simulink model "simulador_secador_solar"  (R2024b)
settings: Solver=VariableStepAuto  StartTime=0.0  StopTime=1000  RelTol=1e-3
values from neighbouring files (symbols this model uses):
  T_mu = 4.5    [G.mat]
settings Model: Creator=Celso  LastModifiedBy=Salvador

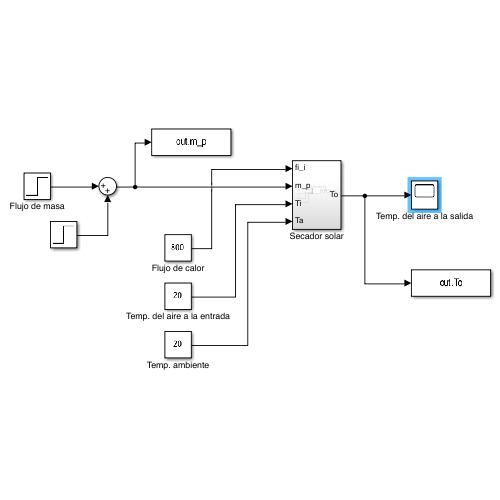
[thumbnail: Simulink's stored preview of the top-level diagram]
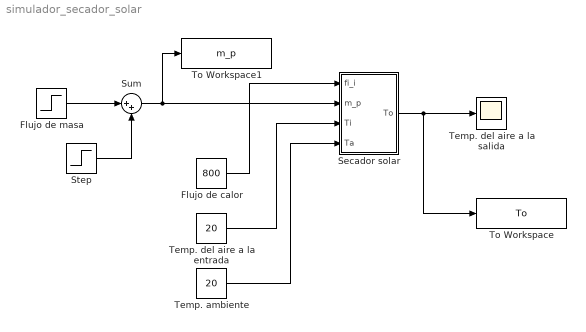
== system simulador_secador_solar ==
  Flujo de calor : Constant  Value=800
  Flujo de masa : Step  Time=0  After=0.02  SampleTime=0
  Secador solar : Subsystem
  Step : Step  Time=450  After=0.03  SampleTime=0
  Sum : Sum  Inputs=|++
  Temp. ambiente : Constant  Value=20
  Temp. del aire a la entrada : Constant  Value=20
  Temp. del aire a la salida : Scope
  To Workspace : ToWorkspace  VariableName=To  SampleTime=T_mu
  To Workspace1 : ToWorkspace  VariableName=m_p  SampleTime=T_mu
  wires:
  Temp. del aire a la entrada/1 -> Secador solar/3(Ti)
  Temp. ambiente/1 -> Secador solar/4(Ta)
  Secador solar/1(To) -> To Workspace/1, Temp. del aire a la salida/1
  Flujo de calor/1 -> Secador solar/1(fi_i)
  Flujo de masa/1 -> Sum/1
  Sum/1 -> To Workspace1/1, Secador solar/2(m_p)
  Step/1 -> Sum/2

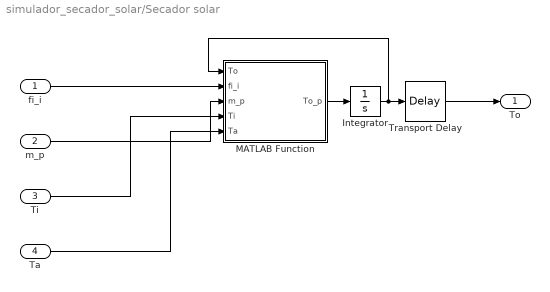
== system simulador_secador_solar/Secador solar ==
  fi_i : Inport
  m_p : Inport  Port=2
  Ti : Inport  Port=3
  Ta : Inport  Port=4
  Integrator : Integrator  InitialCondition=20
  MATLAB Function : MATLAB Function  TreatAsAtomicUnit=on
  Transport Delay : TransportDelay  DelayTime=10  InitialOutput=20
  To : Outport
  wires:
  Integrator/1 -> MATLAB Function/1(To), Transport Delay/1
  MATLAB Function/1(To_p) -> Integrator/1
  fi_i/1 -> MATLAB Function/2(fi_i)
  Ta/1 -> MATLAB Function/5(Ta)
  Ti/1 -> MATLAB Function/4(Ti)
  m_p/1 -> MATLAB Function/3(m_p)
  Transport Delay/1 -> To/1

== matlab function simulador_secador_solar/Secador solar/MATLAB Function ==
  data: To input; To_p output; fi_i input; m_p input; Ti input; Ta input
function To_p = fcn(To,fi_i,m_p,Ti,Ta)

%Simula el calentamiento del aire en un secador solar
%To: temperatura del aire a la salida (°C)
%Ti: temperatura del aire a la entrada (°C)
%V: voltaje aplicado a la resistencia
%   eléctrica del calentador (volt)
%m_p: flujo de masa del aire que ingresa y sale del
%     secador solar (Kg/seg)
%Ta: temperatura ambiente (°C)

M = 0.9; %masa del aire en el secador solar (Kg)
c = 1005; %calor específico del aire (J/Kg-°C)
%fi_i = 800; %Flujo de calor proporcionada por la radiación solar
R = 2; %Resistencia térmica (°C.seg/J)


To_p = fi_i/(M*c) - m_p*(To-Ti)/M - (To-Ta)/(M*c*R)
